simulink model "untitled"  (R2020a)
settings: Solver=FixedStepAuto  StartTime=0.0  StopTime=50  FixedStep=0.001  RelTol=1e-3
libraries: simulink x6
settings Model: Creator=45489  LastModifiedBy=45489

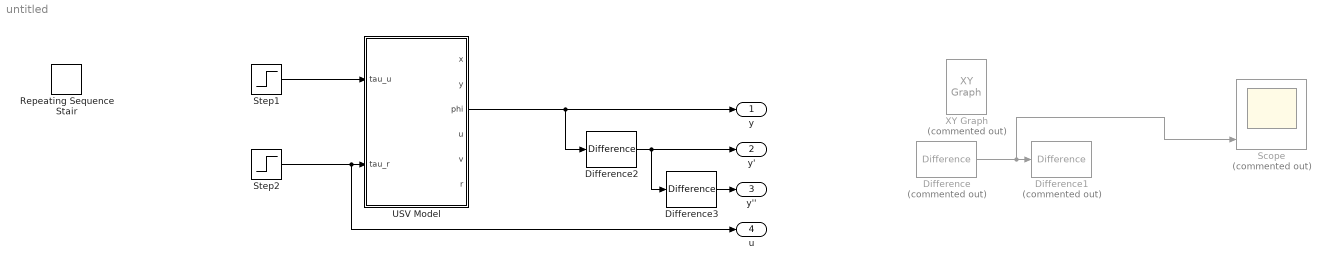
== system untitled ==
  Difference : simulink/Discrete/Difference  Commented=on  ICPrevInput=0.0  OutMin=[]  OutMax=[]  OutDataType=fixdt(1, 16)  OutScaling=2^-10  DoSatur=off
  Difference1 : simulink/Discrete/Difference  Commented=on  ICPrevInput=0.0  OutMin=[]  OutMax=[]  OutDataType=fixdt(1, 16)  OutScaling=2^-10  DoSatur=off
  Difference2 : simulink/Discrete/Difference  ICPrevInput=0.0  OutMin=[]  OutMax=[]  OutDataType=fixdt(1, 16)  OutScaling=2^-10  DoSatur=off
  Difference3 : simulink/Discrete/Difference  ICPrevInput=0.0  OutMin=[]  OutMax=[]  OutDataType=fixdt(1, 16)  OutScaling=2^-10  DoSatur=off
  Repeating Sequence Stair : simulink/Sources/Repeating Sequence Stair  OutValues=[0 1 0 0 0 0 0 ].'  tsamp=20  OutMin=[]  OutMax=[]  OutDataTypeStr=double  OutputDataTypeScalingMode=double  OutDataType=fixdt(0,8)  ConRadixGroup=Best Precision: Vector-wise  OutScaling=2^-12
  Scope : Scope  Commented=on  NumInputPorts=3
  Step1 : Step  SampleTime=0
  Step2 : Step  SampleTime=0
  USV Model : Subsystem
  XY Graph : simulink/Sinks/XY Graph  Commented=on  xmin=-15  xmax=15  ymin=-15  ymax=15  st=0.01
  y : Outport
  y' : Outport  Port=2
  y'' : Outport  Port=3
  u : Outport  Port=4
  wires:
  Step2/1 -> u/1, USV Model/2(tau_r)
  Difference/1 -> Scope/3, Difference1/1
  Step1/1 -> USV Model/1(tau_u)
  USV Model/3(phi) -> Difference2/1, y/1
  Difference2/1 -> Difference3/1, y'/1
  Difference3/1 -> y''/1

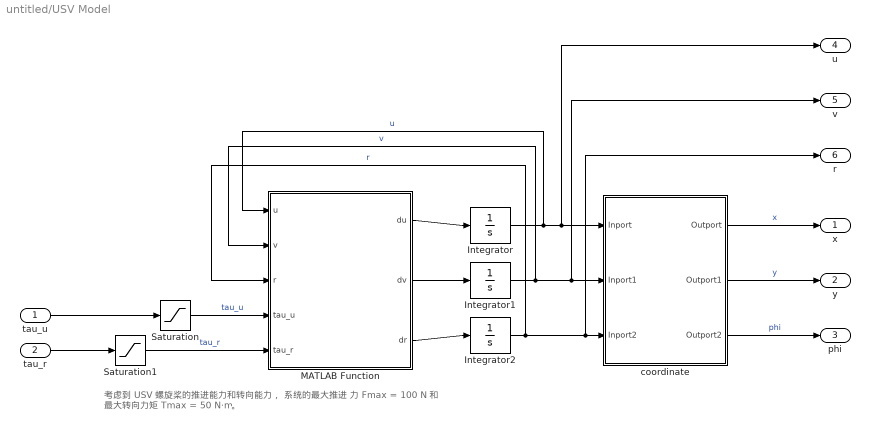
== system untitled/USV Model ==
  note: 考虑到 USV 螺旋桨的推进能力和转向能力，
      | 系统的最大推进 力 Fmax = 100 N 和 最大转向力矩 Tmax = 50 N·m。
  tau_u : Inport
  tau_r : Inport  Port=2
  Integrator : Integrator
  Integrator1 : Integrator
  Integrator2 : Integrator
  MATLAB Function : MATLAB Function  TreatAsAtomicUnit=on
  Saturation : Saturate  UpperLimit=100  LowerLimit=0
  Saturation1 : Saturate  UpperLimit=+50  LowerLimit=-50
  coordinate : Subsystem
  x : Outport
  y : Outport  Port=2
  phi : Outport  Port=3
  u : Outport  Port=4
  v : Outport  Port=5
  r : Outport  Port=6
  wires:
  Saturation/1 -> MATLAB Function/4(tau_u)  "tau_u"
  Integrator/1 -> MATLAB Function/1(u), u/1, coordinate/1(Inport)  "u"
  Integrator1/1 -> MATLAB Function/2(v), v/1, coordinate/2(Inport1)  "v"
  MATLAB Function/3(dr) -> Integrator2/1
  Integrator2/1 -> MATLAB Function/3(r), r/1, coordinate/3(Inport2)  "r"
  MATLAB Function/1(du) -> Integrator/1
  Saturation1/1 -> MATLAB Function/5(tau_r)  "tau_r"
  MATLAB Function/2(dv) -> Integrator1/1
  coordinate/1(Outport) -> x/1  "x"
  tau_r/1 -> Saturation1/1
  tau_u/1 -> Saturation/1
  coordinate/3(Outport2) -> phi/1  "phi"
  coordinate/2(Outport1) -> y/1  "y"

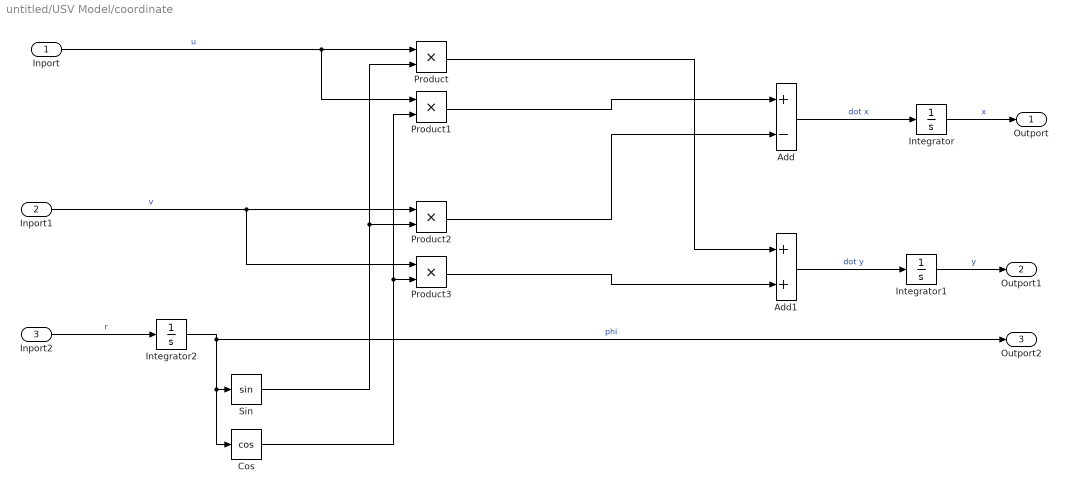
== system untitled/USV Model/coordinate ==
  Inport : Inport
  Inport1 : Inport  Port=2
  Inport2 : Inport  Port=3
  Add : Sum  Inputs=+-
  Add1 : Sum
  Cos : Trigonometry  Operator=cos
  Integrator : Integrator
  Integrator1 : Integrator
  Integrator2 : Integrator
  Product{,1..3} (4 alike) : Product
  Sin : Trigonometry
  Outport : Outport
  Outport1 : Outport  Port=2
  Outport2 : Outport  Port=3
  wires:
  Integrator/1 -> Outport/1  "x"
  Add/1 -> Integrator/1  "dot x"
  Integrator2/1 -> Outport2/1, Cos/1, Sin/1  "phi"
  Product2/1 -> Add/2
  Add1/1 -> Integrator1/1  "dot y"
  Sin/1 -> Product/2, Product2/2
  Cos/1 -> Product1/2, Product3/2
  Inport/1 -> Product1/1, Product/1  "u"
  Product3/1 -> Add1/2
  Inport2/1 -> Integrator2/1  "r"
  Inport1/1 -> Product3/1, Product2/1  "v"
  Product1/1 -> Add/1
  Product/1 -> Add1/1
  Integrator1/1 -> Outport1/1  "y"

== matlab function untitled/USV Model/MATLAB Function ==
  data: u input; du output; v input; r input; tau_u input; tau_r input; dv output; dr output
function [du, dv, dr] = usv(u, v, r, tau_u, tau_r)
    du=0.1*r*2+v*r+tau_u/33-5*u/33;
    dv=50/967*r-10/967*tau_r-5000/31911*v-r*u;
    dr=100/967*tau_r-500/967*r+50/967*v;
